simulink model "failed_model"  (R2020a)
settings: Solver=VariableStepAuto  StartTime=0.0  StopTime=10.0  RelTol=1e-3
undefined symbols (not defined in the file or in its folder): p_dot, q_dot, r_dot
settings Model: Creator=o_belzil  LastModifiedBy=o_belzil

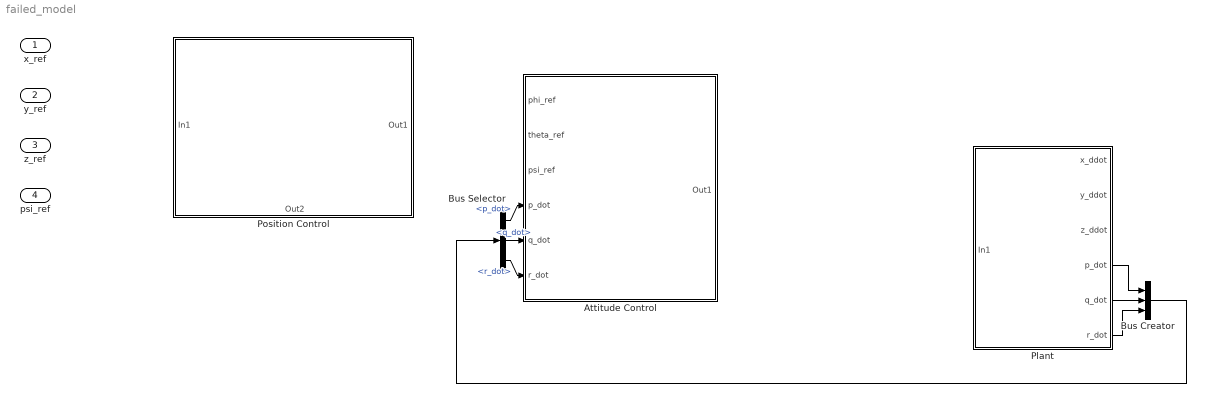
== system failed_model ==
  x_ref : Inport
  y_ref : Inport  Port=2
  z_ref : Inport  Port=3
  psi_ref : Inport  Port=4
  Attitude Control : Subsystem
  Bus Creator : BusCreator  Inputs=p_dot,q_dot,r_dot
  Bus Selector : BusSelector  OutputSignals=p_dot,q_dot,r_dot
  Plant : Subsystem
  Position Control : Subsystem
      settings: PortSchema="{\"entries\":[{\"content\":{\"sides\":[{\"content\":{\"connectorIds\":[\"In1\"]},\"type\":\"ConnectorPlacement.EquallySpacedRectSide\",\"uuid\":\"d7cc4d15-1547-4393-889e-795e986cf8ca\"},{\"content\":{\"connectorIds\":[\"Out1\"],\"side\":\"RIGHT\"},\"type\":\"ConnectorPlacement.EquallySpacedRectSide\",\"uuid\":\"a283f022-b97c-4b70-a869-5d2bb415b2da\"},{\"content\":{\"connectorIds\":[],\"side\":\"TOP\"},\"type\":\"ConnectorPlacement.EquallySpacedRectSide\",\"uuid\":\"b8a7e32b-7c88-4b2a-a1d4-b5daf1c95bb3\"},{\"content\":{\"connectorIds\":[\"Out2\"],\"side\":\"BOTTOM\"},\"type\":\"ConnectorPlacement.EquallySpacedRectSide\",\"uuid\":\"39e324cb-c36e-43a3-8710-9992989a5d33\"}]},\"type\":\"ConnectorPlacement.EquallySpacedConnector\",\"uuid\":\"dcd6118b-c49d-4322-b01a-08a5830d18e4\"}],\"packageUris\":[\"http://schema.mathworks.com/mf0/Connector/19700101\"],\"version\":\"1.0\"}"
  wires:
  Plant/4(p_dot) -> Bus Creator/1
  Plant/5(q_dot) -> Bus Creator/2
  Plant/6(r_dot) -> Bus Creator/3
  Bus Creator/1 -> Bus Selector/1
  Bus Selector/1 -> Attitude Control/4(p_dot)  "<p_dot>"
  Bus Selector/2 -> Attitude Control/5(q_dot)  "<q_dot>"
  Bus Selector/3 -> Attitude Control/6(r_dot)  "<r_dot>"

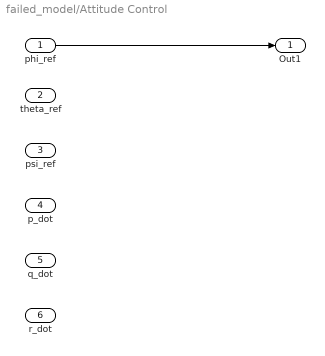
== system failed_model/Attitude Control ==
  phi_ref : Inport
  theta_ref : Inport  Port=2
  psi_ref : Inport  Port=3
  p_dot : Inport  Port=4
  q_dot : Inport  Port=5
  r_dot : Inport  Port=6
  Out1 : Outport
  wires:
  phi_ref/1 -> Out1/1

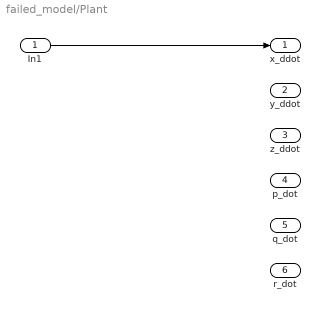
== system failed_model/Plant ==
  In1 : Inport
  x_ddot : Outport
  y_ddot : Outport  Port=2
  z_ddot : Outport  Port=3
  p_dot : Outport  Port=4
  q_dot : Outport  Port=5
  r_dot : Outport  Port=6
  wires:
  In1/1 -> x_ddot/1

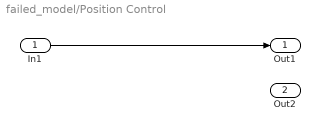
== system failed_model/Position Control ==
  In1 : Inport
  Out1 : Outport
  Out2 : Outport  Port=2
  wires:
  In1/1 -> Out1/1
